simulink model "verify_layerwall_static_mdl"  (R2016b)
settings: Solver=ode45  StartTime=0.0  StopTime=10*24*3600  MaxStep=600  RelTol=1e-3  EnableMultiTasking=on
libraries: carnot x1
settings Model: Creator=drhf  LastModifiedBy=drhf
settings DataIOCC: LimitDataPoints=on  SaveFormat=Array
settings OptimizationCC: DefaultParameterBehavior=Inlined  LifeSpan=inf
settings DebuggingCC: UnderspecifiedInitializationDetection=Classic  MergeDetectMultiDrivingBlocksExec=none  SolverPrmCheckMsg=warning  SFUnexpectedBacktrackingDiag=warning  SFNoUnconditionalDefaultTransitionDiag=warning  SFExecutionAtInitializationDiag=none
settings HardwareCC: ProdBitPerPointer=32  ProdBitPerSizeT=32  ProdBitPerPtrDiffT=32  ProdLargestAtomicFloat=None  ProdIntDivRoundTo=Undefined  ProdEndianess=Unspecified  ProdWordSize=32  ProdHWDeviceType=32-bit Generic
settings ModelReferenceCC: PropagateSignalLabelsOutOfModel=off
settings GRTTargetCC: TargetLangStandard=C89/C90 (ANSI)  GeneratePreprocessorConditionals=Disable all
settings ConfigComp: CovMetricSettings=dw  CovHtmlReporting=on  CovSaveCumulativeToWorkspaceVar=on  CovSaveSingleToWorkspaceVar=on  CovExternalEMLEnable=off

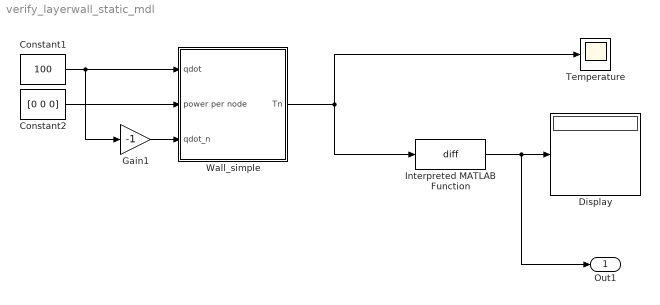
== system verify_layerwall_static_mdl ==
  Constant1 : Constant  Value=100
  Constant2 : Constant  Value=[0 0 0]
  Display : Display
  Gain1 : Gain  Gain=-1
  Interpreted MATLAB Function : MATLABFcn  MATLABFcn=diff
  Temperature : Scope
  Wall_simple : Subsystem  mask(simplified wall){wallsize=[1 1], d=[0.1 0.1 0.1], cond=[1 1 1], cwall=[0.28 0.28 0.28]*3600, rho=[2000 200 2000], emission_in=.96, dactive=[0.075 0.15 0.225], t0=0, tau=1*3600}
      mask prompts: wallsize "size of wall [m] [height width]"; d "thickness of layers [m] (vector) (0 = towards this room)"; cond "conductivity of layers [W/(m*K)] (vector)"; cwall "capacity of layers [J/(kg*K)] (vector)"; rho "density of layers [kg/m³]"; emission_in "emission of wall surface"; dactive "depth active layer in m from inner surface  (-1 = none)"; t0 "initial temperature [degree centigrade]"; tau "time-constant of wall [s]"
      mask help: simplified model to test wall_basic
      mask init:
      | position = [0 90 0 ];
      | % nodes = length(d);
      | wallheight = wallsize(1);
      | wallsurface = wallsize(1)*wallsize(2);
      | 
      | if (dactive>=0) 
      |     active = 1;
      | else
      |     active = 0;
      | end
  Out1 : Outport
  wires:
  Constant2/1 -> Wall_simple/2(power per node)
  Constant1/1 -> Gain1/1, Wall_simple/1(qdot)
  Gain1/1 -> Wall_simple/3(qdot_n)
  Wall_simple/1(Tn) -> Interpreted MATLAB Function/1, Temperature/1
  Interpreted MATLAB Function/1 -> Out1/1, Display/1

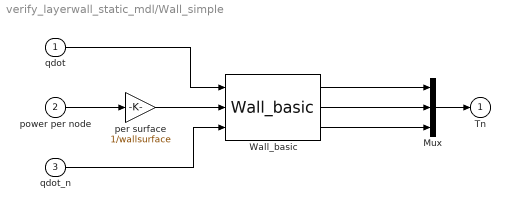
== system verify_layerwall_static_mdl/Wall_simple ==
  qdot : Inport
  power per node : Inport  Port=2
  qdot_n : Inport  Port=3
  Mux : Mux  Inputs=3
  Wall_basic : carnot/Basic/Thermal_Models/Wall_basic  tau=tau  t0=t0  d=d  dactive=dactive  cond=cond  cwall=cwall  rho=rho
  per surface : Gain  Gain=1/wallsurface  SaturateOnIntegerOverflow=on  OutDataTypeStr=Inherit: Same as input  ParamDataTypeStr=Inherit: Same as input
  Tn : Outport
  wires:
  power per node/1 -> per surface/1
  per surface/1 -> Wall_basic/2
  Wall_basic/1 -> Mux/1
  Wall_basic/3 -> Mux/3
  Wall_basic/2 -> Mux/2
  Mux/1 -> Tn/1
  qdot/1 -> Wall_basic/1
  qdot_n/1 -> Wall_basic/3
